simulink model "sim_Ex6"  (R2022b)
settings: Solver=FixedStepAuto  StartTime=0.0  StopTime=10.0  FixedStep=1e-3
values from neighbouring files (symbols this model uses):
  Freq = freq(i)    [sim_Ex6_script.m]
libraries: spsParallelRLCBranchLib x2, spsControlledVoltageSourceLib x1, spsVoltageMeasurementLib x1, sps_lib x1
settings Model: Creator=MAAM  LastModifiedBy=MAAM

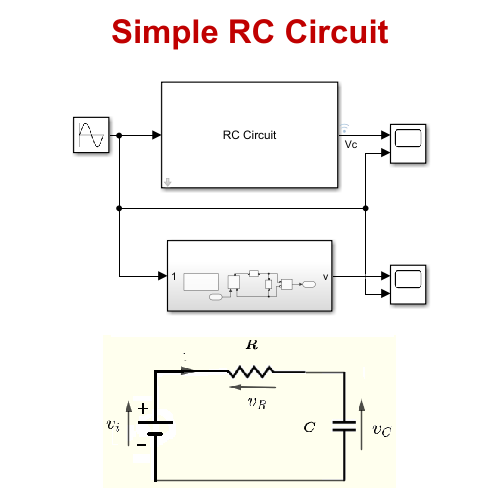
[thumbnail: Simulink's stored preview of the top-level diagram]
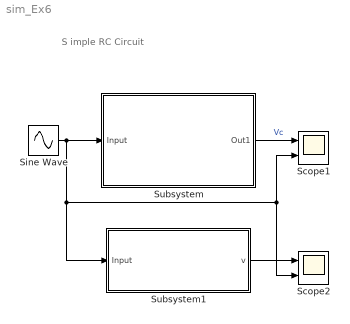
== system sim_Ex6 ==
  note: S imple RC Circuit
  Scope1 : Scope  NumInputPorts=2
  Scope2 : Scope  NumInputPorts=2
  Sine Wave : Sin  Amplitude=5  Frequency=2*pi*Freq  SampleTime=0
  Subsystem : Subsystem  mask{R=1500, C=1e-3}
      mask prompts: R "Resistance (Ohms)R"; C "Capacitance (F)"
      mask Display: fprintf('RC Circuit');
  Subsystem1 : Subsystem
  wires:
  Sine Wave/1 -> Scope1/2, Scope2/2, Subsystem1/1(Input), Subsystem/1(Input)
  Subsystem/1(Out1) -> Scope1/1  "Vc"
  Subsystem1/1(v) -> Scope2/1

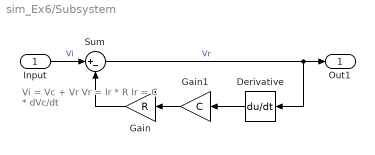
== system sim_Ex6/Subsystem ==
  note: Vi = Vc + Vr
      | Vr = Ir * R
      | Ir = C * dVc/dt
  Input : Inport
  Derivative : Derivative
  Gain : Gain  Gain=R
  Gain1 : Gain  Gain=C
  Sum : Sum  Inputs=|+-
  Out1 : Outport
  wires:
  Input/1 -> Sum/1  "Vi"
  Gain/1 -> Sum/2
  Sum/1 -> Out1/1, Derivative/1  "Vr"
  Derivative/1 -> Gain1/1
  Gain1/1 -> Gain/1

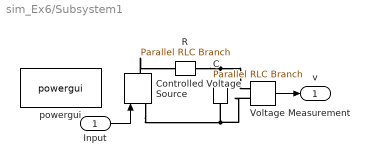
== system sim_Ex6/Subsystem1 ==
  Input : Inport
  C : spsParallelRLCBranchLib/Parallel RLC Branch  LConnTagsString=a  RConnTagsString=__new0  BranchType=C  Resistance=inf  Inductance=inf  SetiL0=off  InitialCurrent=0  Capacitance=1e-3  Setx0=off  InitialVoltage=0  Measurements=None
  Controlled Voltage Source : spsControlledVoltageSourceLib/Controlled Voltage Source  Initialize=on  Source_Type=AC  Amplitude=0  Phase=0  Frequency=0  Measurements=None
  R : spsParallelRLCBranchLib/Parallel RLC Branch  LConnTagsString=a  RConnTagsString=__new0  BranchType=R  Resistance=1500  Inductance=inf  SetiL0=off  InitialCurrent=0  Capacitance=1e-3  Setx0=off  InitialVoltage=0  Measurements=None
  Voltage Measurement : spsVoltageMeasurementLib/Voltage Measurement  PhasorSimulation=off  OutputType=Complex  PSBequivalent=0
  powergui : sps_lib/powergui  Priority=1  SimulationMode=Continuous  SampleTime=50e-6  frequency=60  Iterations=50  frequencyindice=0  Pbase=100e6  ErrMax=1e-4  UnitsV=kV  UnitsW=MW  buscounter=0  FunctionMessages=off  echomessages=off  EnableUseOfTLC=off  CurrentSourceSwitches=off  DisableSnubberDevices=off  DisableRonSwitches=off  DisableVfSwitches=off  DisplayEquations=off  AutomaticDiscreteSolvers=off  SolverType=Tustin/Backward Euler (TBE)  Interpol=off  ExternalGateDelay=off  methode=off  Ts=100  x0status=blocks  SPID=on  SwTol=0  HookPort=off  NonlinearTolerance=1e-4  nMaxIteration=100  ContinueOnMaxIteration=off  RestoreLinks=warning  ResistiveCurrentMeasurement=off  Frange=[0:2:500]  Ylog=off  Xlog=on  ShowGrid=off  save=off  variable=ZData  structure=0  ZoomFFT=off  StartTime=0.0  cycles=1  DisplayStyle=1  fundamental=60  FreqAxis=off  MaxFrequency=1000  frequencyindicesteady=1  RmsSteady=1  display=off
  v : Outport
  wires:
  Voltage Measurement/1 -> v/1
  Input/1 -> Controlled Voltage Source/1
  connections:
  R/RConn1 -- C/LConn1 -- Voltage Measurement/LConn1
  Voltage Measurement/LConn2 -- Controlled Voltage Source/LConn1 -- C/RConn1
  Controlled Voltage Source/RConn1 -- R/LConn1
